simulink model "input_model"  (R2022b)
settings: Solver=VariableStepAuto  StartTime=0.0  StopTime=24*3600  RelTol=1e-3
settings Model: Creator=egidi  LastModifiedBy=egidi

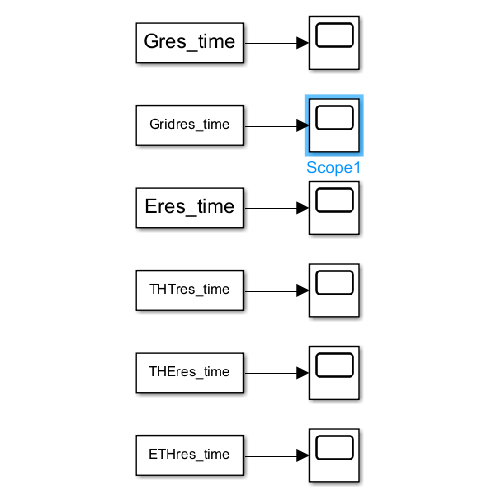
[thumbnail: Simulink's stored preview of the top-level diagram]
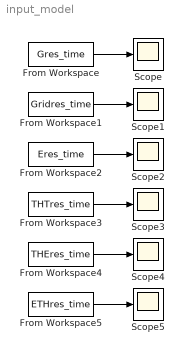
== system input_model ==
  From Workspace : FromWorkspace  VariableName=Gres_time
  From Workspace1 : FromWorkspace  VariableName=Gridres_time
  From Workspace2 : FromWorkspace  VariableName=Eres_time
  From Workspace3 : FromWorkspace  VariableName=THTres_time
  From Workspace4 : FromWorkspace  VariableName=THEres_time
  From Workspace5 : FromWorkspace  VariableName=ETHres_time
  Scope{,1..5} (6 alike) : Scope
  wires:
  From Workspace/1 -> Scope/1
  From Workspace1/1 -> Scope1/1
  From Workspace2/1 -> Scope2/1
  From Workspace3/1 -> Scope3/1
  From Workspace4/1 -> Scope4/1
  From Workspace5/1 -> Scope5/1
